simulink model "FlexLoadControl"  (R2019a)
settings: Solver=ode4  StartTime=0.0  StopTime=1  FixedStep=1e-4  MaxStep=1e-4  MinStep=1e-6  RelTol=1e-10
InitFcn:
  | Rs = 0.011
  | Ld = 0.018
  | Lq = 0.018
  | Fi = 0.055
  | p = 4
  | J = 0.102
  | b = 0.18
  | 
  | A1 = 1
  | B1 = -5000
  | B2 = -0.0200
  | B3 = 10
  | C1 = 500
  | C2 = -2.499999800000000e+04
  | C3 = -90.999999999999990
  | C4 = 110
  | 
  | tC = 10
  | kk1 = -1011
  | kk2 = -241.5
  | kk3 = -20
  | k3 = -1.620402364619914
  | k4 = -0.507865883970218
  | k5 = -0.507865883970218
  | k6 = -0.294132929497733
  | 
  | x1e = 0
  | x2e = 0
  | x3e = 0
  | ide = 3.024305555555556
  | iqe = 0.307424053403619
  | 
  | tO = 20
  | g1 = 0.164052784000000
  | g2 = -2.996000000000000
  | g3 = 8.089800000000000e+02
settings Model: Creator=LiLid  LastModifiedBy=LiLid

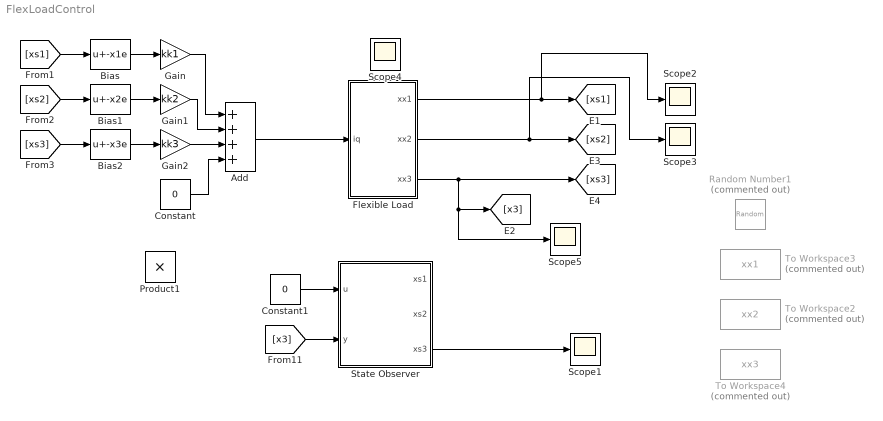
== system FlexLoadControl ==
  Add : Sum  Inputs=++++
  Bias : Bias  Bias=-x1e
  Bias1 : Bias  Bias=-x2e
  Bias2 : Bias  Bias=-x3e
  Constant : Constant  Value=0
  Constant1 : Constant  Value=0
  Flexible Load : Subsystem
  Gain : Gain  Gain=kk1
  Gain1 : Gain  Gain=kk2
  Gain2 : Gain  Gain=kk3
  Product1 : Product
  Random Number1 : RandomNumber  Commented=on  Variance=0.1  SampleTime=0.0001
  Scope{1..5} (5 alike) : Scope
  State Observer : Subsystem
  To Workspace2 : ToWorkspace  Commented=on  VariableName=xx2  SampleTime=-1
      settings: Save2DSignal=2-D array (concatenate along first dimension)
  To Workspace3 : ToWorkspace  Commented=on  VariableName=xx1  SampleTime=-1
      settings: Save2DSignal=2-D array (concatenate along first dimension)
  To Workspace4 : ToWorkspace  Commented=on  VariableName=xx3  SampleTime=-1
      settings: Save2DSignal=2-D array (concatenate along first dimension)
  wires:
  Flexible Load/3(xx3) -> Scope5/1, [x3], [xs3]
  State Observer/3(xs3) -> Scope1/1
  [xs1] -> Bias/1
  [xs2] -> Bias1/1
  [xs3] -> Bias2/1
  Bias/1 -> Gain/1
  Gain/1 -> Add/1
  Bias1/1 -> Gain1/1
  Gain1/1 -> Add/2
  Bias2/1 -> Gain2/1
  Gain2/1 -> Add/3
  Flexible Load/2(xx2) -> [xs2], Scope3/1
  [x3] -> State Observer/2(y)
  Constant1/1 -> State Observer/1(u)
  Flexible Load/1(xx1) -> Scope2/1, [xs1]
  Constant/1 -> Add/4
  Add/1 -> Flexible Load/1(iq)

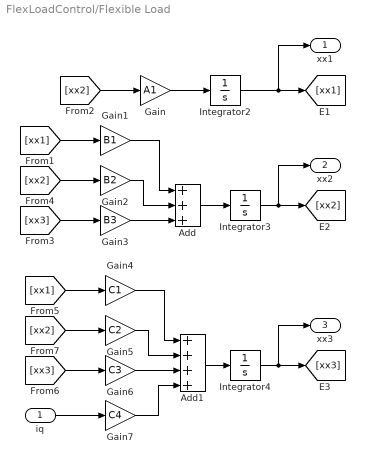
== system FlexLoadControl/Flexible Load ==
  iq : Inport
  Add : Sum  Inputs=+++
  Add1 : Sum  Inputs=++++
  Gain : Gain  Gain=A1
  Gain1 : Gain  Gain=B1
  Gain2 : Gain  Gain=B2
  Gain3 : Gain  Gain=B3
  Gain4 : Gain  Gain=C1
  Gain5 : Gain  Gain=C2
  Gain6 : Gain  Gain=C3
  Gain7 : Gain  Gain=C4
  Integrator2 : Integrator  InitialCondition=2.5e-3
  Integrator3 : Integrator
  Integrator4 : Integrator  InitialCondition=1.2
  xx1 : Outport
  xx2 : Outport  Port=2
  xx3 : Outport  Port=3
  wires:
  Integrator2/1 -> xx1/1, [xx1]
  Integrator3/1 -> [xx2], xx2/1
  Integrator4/1 -> xx3/1, [xx3]
  [xx2] -> Gain/1
  Gain/1 -> Integrator2/1
  [xx1] -> Gain1/1
  [xx2] -> Gain2/1
  [xx3] -> Gain3/1
  Add/1 -> Integrator3/1
  Gain3/1 -> Add/3
  Gain2/1 -> Add/2
  Gain1/1 -> Add/1
  [xx1] -> Gain4/1
  [xx2] -> Gain5/1
  Add1/1 -> Integrator4/1
  Gain5/1 -> Add1/2
  [xx3] -> Gain6/1
  Gain6/1 -> Add1/3
  Gain4/1 -> Add1/1
  iq/1 -> Gain7/1
  Gain7/1 -> Add1/4

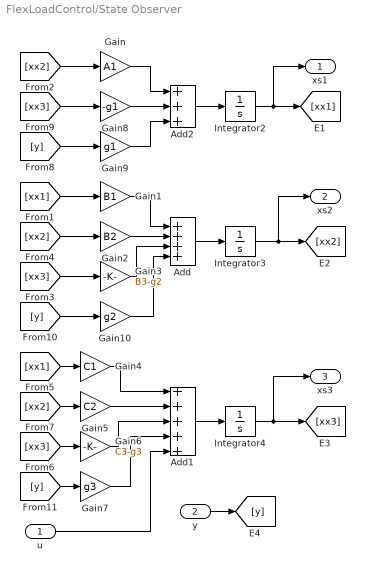
== system FlexLoadControl/State Observer ==
  u : Inport
  y : Inport  Port=2
  Add : Sum  Inputs=++++
  Add1 : Sum  Inputs=+++++
  Add2 : Sum  Inputs=+++
  Gain : Gain  Gain=A1
  Gain1 : Gain  Gain=B1
  Gain10 : Gain  Gain=g2
  Gain2 : Gain  Gain=B2
  Gain3 : Gain  Gain=B3-g2
  Gain4 : Gain  Gain=C1
  Gain5 : Gain  Gain=C2
  Gain6 : Gain  Gain=C3-g3
  Gain7 : Gain  Gain=g3
  Gain8 : Gain  Gain=-g1
  Gain9 : Gain  Gain=g1
  Integrator2 : Integrator
  Integrator3 : Integrator
  Integrator4 : Integrator
  xs1 : Outport
  xs2 : Outport  Port=2
  xs3 : Outport  Port=3
  wires:
  Integrator3/1 -> [xx2], xs2/1
  Integrator4/1 -> [xx3], xs3/1
  [xx2] -> Gain/1
  [xx1] -> Gain1/1
  [xx2] -> Gain2/1
  [xx3] -> Gain3/1
  Add/1 -> Integrator3/1
  Gain3/1 -> Add/3
  Gain2/1 -> Add/2
  Gain1/1 -> Add/1
  [xx1] -> Gain4/1
  [xx2] -> Gain5/1
  Add1/1 -> Integrator4/1
  Gain5/1 -> Add1/2
  [xx3] -> Gain6/1
  Gain6/1 -> Add1/3
  Gain4/1 -> Add1/1
  Gain7/1 -> Add1/4
  y/1 -> [y]
  [xx3] -> Gain8/1
  [y] -> Gain9/1
  Gain8/1 -> Add2/2
  Gain9/1 -> Add2/3
  Gain/1 -> Add2/1
  Add2/1 -> Integrator2/1
  Integrator2/1 -> xs1/1, [xx1]
  Gain10/1 -> Add/4
  [y] -> Gain10/1
  [y] -> Gain7/1
  u/1 -> Add1/5
